simulink model "partB"  (R2018b)
settings: Solver=VariableStepAuto  StartTime=0.0  StopTime=10.0  RelTol=1e-3
settings Model: Creator=amir  LastModifiedBy=amir

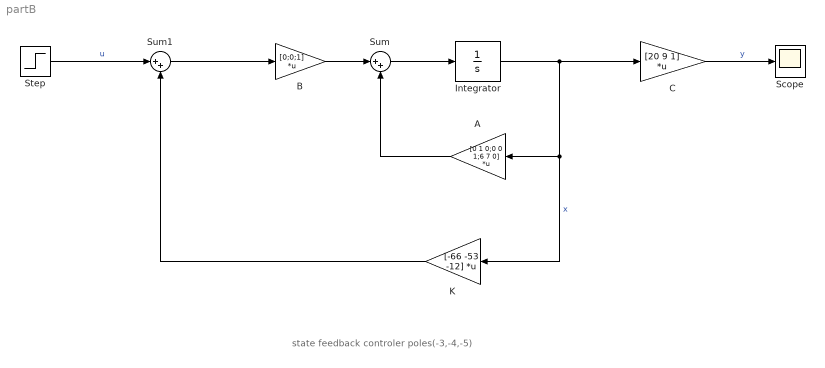
== system partB ==
  note: state feedback controler
      | poles(-3,-4,-5)
  A : Gain  Gain=[0 1 0;0 0 1;6 7 0]  Multiplication=Matrix(K*u) (u vector)
  B : Gain  Gain=[0;0;1]  Multiplication=Matrix(K*u) (u vector)
  C : Gain  Gain=[20 9 1]  Multiplication=Matrix(K*u) (u vector)
  Integrator : Integrator  InitialCondition=[1;1;1]
  K : Gain  Gain=[-66 -53 -12]  Multiplication=Matrix(K*u) (u vector)
  Scope : Scope
  Step : Step  SampleTime=0
  Sum : Sum  Inputs=|++
  Sum1 : Sum  Inputs=|++
  wires:
  K/1 -> Sum1/2
  Sum1/1 -> B/1
  C/1 -> Scope/1  "y"
  Integrator/1 -> K/1, A/1, C/1  "x"
  B/1 -> Sum/1
  A/1 -> Sum/2
  Sum/1 -> Integrator/1
  Step/1 -> Sum1/1  "u"
